simulink model "PMSM_S"  (R2023a)
settings: Solver=VariableStepAuto  StartTime=0.0  StopTime=10000  RelTol=1e-3
values from neighbouring files (symbols this model uses):
  i1qn = 1    [PMSM_M.m]
  Jc = 1    [PMSM_M.m]
  Kr_i1d = 1    [PMSM_M.m]
  Kr_i1q = 1    [PMSM_M.m]
  Kr_phi = 1    [PMSM_M.m]
  Kr_w = 1    [PMSM_M.m]
  L1 = 1    [PMSM_M.m]
  Psi = 1    [PMSM_M.m]
  R1 = 1    [PMSM_M.m]
  Ti_i1d = 1    [PMSM_M.m]
  Ti_i1q = 1    [PMSM_M.m]
  Ti_phi = 1    [PMSM_M.m]
  Ti_w = 1    [PMSM_M.m]
  wn = 1    [PMSM_M.m]
settings Model: Creator=samof  LastModifiedBy=samof

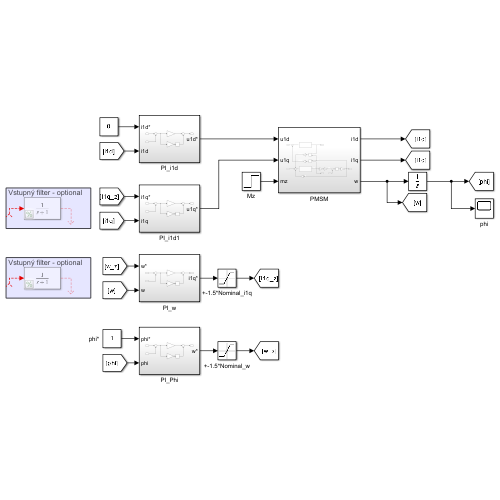
[thumbnail: Simulink's stored preview of the top-level diagram]
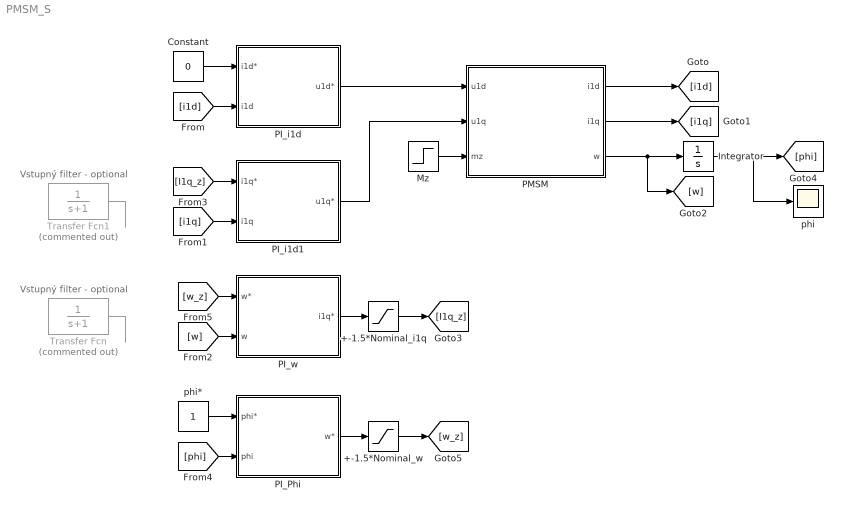
== system PMSM_S ==
  note: Vstupný filter - optional
  note: Vstupný filter - optional
  +-1.5*Nominal_i1q : Saturate  UpperLimit=1.5*i1qn  LowerLimit=-1.5*i1qn
  +-1.5*Nominal_w : Saturate  UpperLimit=1.5*wn  LowerLimit=-1.5*wn
  Constant : Constant  Value=0
  Integrator : Integrator
  Mz : Step  SampleTime=0
  PI_Phi : Subsystem
  PI_i1d : Subsystem
  PI_i1d1 : Subsystem
  PI_w : Subsystem
  PMSM : Subsystem
  Transfer Fcn : TransferFcn  Commented=on  Denominator=[1 1]
  Transfer Fcn1 : TransferFcn  Commented=on  Denominator=[1 1]
  phi : Scope
  phi* : Constant
  wires:
  PMSM/1(i1d) -> [i1d]
  PMSM/2(i1q) -> [i1q]
  [i1d] -> PI_i1d/2(i1d)
  PI_i1d/1(u1d*) -> PMSM/1(u1d)
  [i1q] -> PI_i1d1/2(i1q)
  PI_i1d1/1(u1q*) -> PMSM/2(u1q)
  Constant/1 -> PI_i1d/1(i1d*)
  PI_w/1(i1q*) -> +-1.5*Nominal_i1q/1
  Transfer Fcn/1 -> ?
  ? -> Transfer Fcn/1
  PMSM/3(w) -> [w], Integrator/1
  Integrator/1 -> [phi], phi/1
  [w] -> PI_w/2(w)
  ? -> Transfer Fcn1/1
  Transfer Fcn1/1 -> ?
  [I1q_z] -> PI_i1d1/1(i1q*)
  +-1.5*Nominal_i1q/1 -> [I1q_z]
  PI_Phi/1(w*) -> +-1.5*Nominal_w/1
  [phi] -> PI_Phi/2(phi)
  phi*/1 -> PI_Phi/1(phi*)
  [w_z] -> PI_w/1(w*)
  +-1.5*Nominal_w/1 -> [w_z]
  Mz/1 -> PMSM/3(mz)

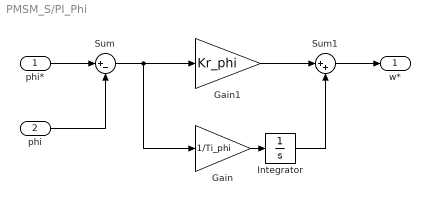
== system PMSM_S/PI_Phi ==
  phi* : Inport
  phi : Inport  Port=2
  Gain : Gain  Gain=1/Ti_phi
  Gain1 : Gain  Gain=Kr_phi
  Integrator : Integrator
  Sum : Sum  Inputs=|+-
  Sum1 : Sum  Inputs=|++
  w* : Outport
  wires:
  phi*/1 -> Sum/1
  phi/1 -> Sum/2
  Gain/1 -> Integrator/1
  Sum1/1 -> w*/1
  Integrator/1 -> Sum1/2
  Sum/1 -> Gain/1, Gain1/1
  Gain1/1 -> Sum1/1

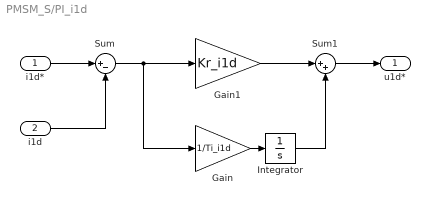
== system PMSM_S/PI_i1d ==
  i1d* : Inport
  i1d : Inport  Port=2
  Gain : Gain  Gain=1/Ti_i1d
  Gain1 : Gain  Gain=Kr_i1d
  Integrator : Integrator
  Sum : Sum  Inputs=|+-
  Sum1 : Sum  Inputs=|++
  u1d* : Outport
  wires:
  i1d*/1 -> Sum/1
  i1d/1 -> Sum/2
  Gain/1 -> Integrator/1
  Sum1/1 -> u1d*/1
  Integrator/1 -> Sum1/2
  Sum/1 -> Gain/1, Gain1/1
  Gain1/1 -> Sum1/1

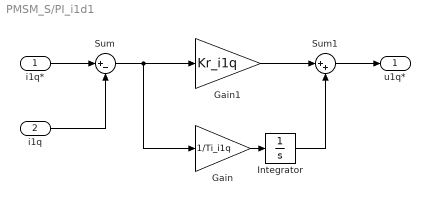
== system PMSM_S/PI_i1d1 ==
  i1q* : Inport
  i1q : Inport  Port=2
  Gain : Gain  Gain=1/Ti_i1q
  Gain1 : Gain  Gain=Kr_i1q
  Integrator : Integrator
  Sum : Sum  Inputs=|+-
  Sum1 : Sum  Inputs=|++
  u1q* : Outport
  wires:
  i1q*/1 -> Sum/1
  i1q/1 -> Sum/2
  Gain/1 -> Integrator/1
  Sum1/1 -> u1q*/1
  Integrator/1 -> Sum1/2
  Sum/1 -> Gain/1, Gain1/1
  Gain1/1 -> Sum1/1

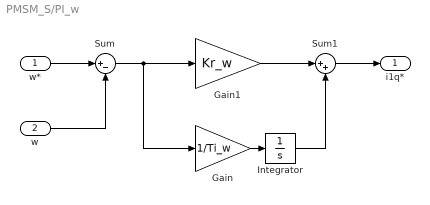
== system PMSM_S/PI_w ==
  w* : Inport
  w : Inport  Port=2
  Gain : Gain  Gain=1/Ti_w
  Gain1 : Gain  Gain=Kr_w
  Integrator : Integrator
  Sum : Sum  Inputs=|+-
  Sum1 : Sum  Inputs=|++
  i1q* : Outport
  wires:
  w*/1 -> Sum/1
  w/1 -> Sum/2
  Gain/1 -> Integrator/1
  Sum1/1 -> i1q*/1
  Integrator/1 -> Sum1/2
  Sum/1 -> Gain/1, Gain1/1
  Gain1/1 -> Sum1/1

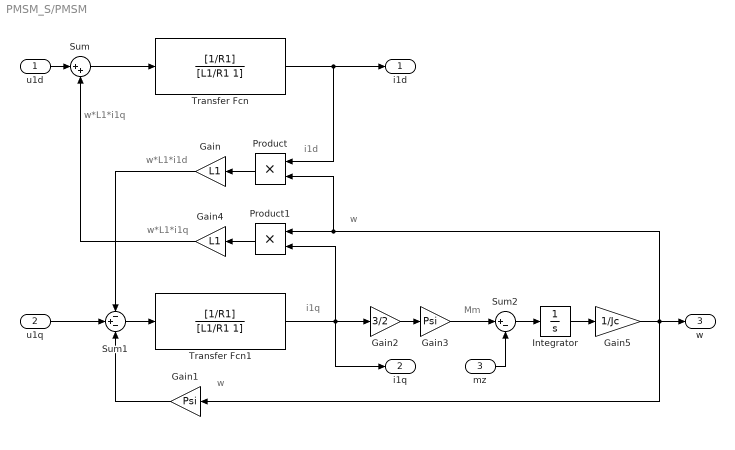
== system PMSM_S/PMSM ==
  note: Mm
  note: i1d
  note: w*L1*i1q
  note: w*L1*i1d
  note: w
  note: i1q
  note: w*L1*i1q
  note: w
  u1d : Inport
  u1q : Inport  Port=2
  mz : Inport  Port=3
  Gain : Gain  Gain=L1
  Gain1 : Gain  Gain=Psi
  Gain2 : Gain  Gain=3/2
  Gain3 : Gain  Gain=Psi
  Gain4 : Gain  Gain=L1
  Gain5 : Gain  Gain=1/Jc
  Integrator : Integrator
  Product : Product
  Product1 : Product
  Sum : Sum  Inputs=|++
  Sum1 : Sum  Inputs=-+-
  Sum2 : Sum  Inputs=|+-
  Transfer Fcn : TransferFcn  Numerator=[1/R1]  Denominator=[L1/R1 1]
  Transfer Fcn1 : TransferFcn  Numerator=[1/R1]  Denominator=[L1/R1 1]
  i1d : Outport
  i1q : Outport  Port=2
  w : Outport  Port=3
  wires:
  u1d/1 -> Sum/1
  Gain4/1 -> Sum/2
  Sum/1 -> Transfer Fcn/1
  Transfer Fcn/1 -> i1d/1, Product/1
  u1q/1 -> Sum1/2
  Gain/1 -> Sum1/1
  Product/1 -> Gain/1
  Gain1/1 -> Sum1/3
  Gain5/1 -> w/1, Product1/1, Product/2, Gain1/1
  Sum1/1 -> Transfer Fcn1/1
  Transfer Fcn1/1 -> Product1/2, Gain2/1, i1q/1
  Gain2/1 -> Gain3/1
  Gain3/1 -> Sum2/1
  Product1/1 -> Gain4/1
  mz/1 -> Sum2/2
  Sum2/1 -> Integrator/1
  Integrator/1 -> Gain5/1
